simulink model "test"  (R2015a)
settings: Solver=ode1  StartTime=0.0  StopTime=10  FixedStep=0.001  RelTol=1e-3
PostLoadFcn:
  | , if any(exist('dsrtsu_mdlpostloadfcn', 'file') == [2, 3, 6]), try dsrtsu_mdlpostloadfcn('Execute', bdroot); catch fprintf('Error in PostLoadFcn (dsrtsu_mdlpostloadfcn) for model "%s":\n %s\n', bdroot, lasterr); end, end,
values from neighbouring files (symbols this model uses):
  c = rectangle('Parent',ax)    [DoublePendulum.m]    (also in init.m = 2.99880047981; interpolate.m = 2.99880047981; plot_17.m = 2.99880047981)
  g = 9.81    [init.m]    (also in interpolate.m; plot_17.m; plot_generic.m)
  T1 = 0.0395    [init.m]    (also in interpolate.m = 0.025; plot_17.m = 0.025; plot_generic.m)
settings Model: DSRTSU_INTERNAL_RTI_VER=360  DSRTSU_INTERNAL_RTI_TYPE=rti1104  CovSFcnEnable=off  Creator=labor  LastModifiedBy=Schuettler
settings DataIOCC: SignalLoggingSaveFormat=ModelDataLogs
settings OptimizationCC: BlockReduction=off  OptimizeBlockIOStorage=off  BufferReuse=off  GlobalBufferReuse=off  ExpressionFolding=off  ExpressionDepthLimit=2147483647  LocalBlockOutputs=off  InitFltsAndDblsToZero=on  OptimizeModelRefInitCode=on  LifeSpan=1
settings DebuggingCC: UnderspecifiedInitializationDetection=Classic  MergeDetectMultiDrivingBlocksExec=none  SolverPrmCheckMsg=warning  FcnCallInpInsideContextMsg=UseLocalSettings  StateNameClashWarn=warning
settings HardwareCC: ProdIntDivRoundTo=Zero  ProdEndianess=BigEndian  ProdHWDeviceType=Generic->Custom  TargetIntDivRoundTo=Zero  TargetEndianess=BigEndian  TargetHWDeviceType=Generic->Custom
settings RTWCC: SystemTargetFile=ert.tlc  TemplateMakefile=ert_default_tmf  Description=Embedded Coder
settings CodeAppCC: IgnoreCustomStorageClasses=off
settings ERTTargetCC: ParMdlRefBuildCompliant=on  CompOptLevelCompliant=on  ConcurrentExecutionCompliant=on  ERTFirstTimeCompliant=on  SupportContinuousTime=off  SupportVariableSizeSignals=off  ModelStepFunctionPrototypeControlCompliant=on  CPPClassGenCompliant=on  InlinedParameterPlacement=Hierarchical  ERTCustomFileTemplate=example_file_process.tlc

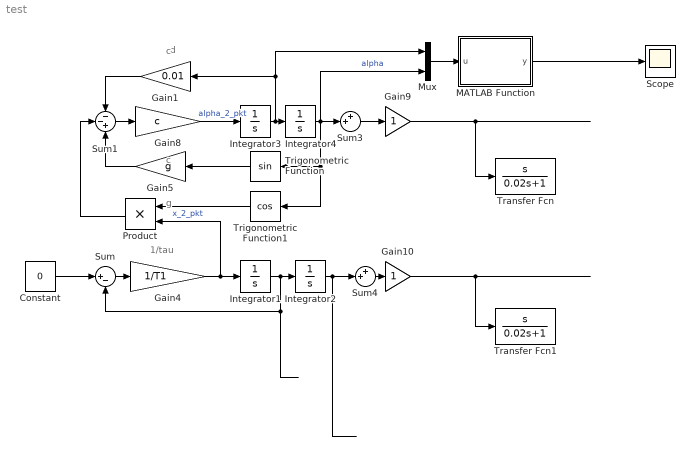
== system test ==
  note: d
  note: 1/tau
  note: g
  note: c
  note: c
  Constant : Constant  Value=0
  Gain1 : Gain  Gain=0.01
  Gain10 : Gain
  Gain4 : Gain  Gain=1/T1
  Gain5 : Gain  Gain=g
  Gain8 : Gain  Gain=c
  Gain9 : Gain
  Integrator1 : Integrator
  Integrator2 : Integrator
  Integrator3 : Integrator
  Integrator4 : Integrator  InitialCondition=2
  MATLAB Function : MATLAB Function  TreatAsAtomicUnit=on
  Mux : Mux  Inputs=2
  Product : Product  RndMeth=Zero
  Scope : Scope
      settings: SaveName=E
  Sum : Sum  Inputs=|+-
  Sum1 : Sum  Inputs=--+
  Sum3 : Sum  Inputs=++|
  Sum4 : Sum  Inputs=++|
  Transfer Fcn : TransferFcn  Numerator=[1 0]  Denominator=[0.02 1]
  Transfer Fcn1 : TransferFcn  Numerator=[1 0]  Denominator=[0.02 1]
  Trigonometric Function : Trigonometry
  Trigonometric Function1 : Trigonometry  Operator=cos
  wires:
  Sum3/1 -> Gain9/1
  Gain9/1 -> Transfer Fcn/1
  Gain10/1 -> Transfer Fcn1/1
  Sum4/1 -> Gain10/1
  Integrator1/1 -> Integrator2/1, Sum/2
  Integrator3/1 -> Gain1/1, Mux/1, Integrator4/1
  Gain4/1 -> Integrator1/1, Product/2  "x_2_pkt"
  Sum/1 -> Gain4/1
  Trigonometric Function1/1 -> Product/1
  Sum1/1 -> Gain8/1
  Gain8/1 -> Integrator3/1  "alpha_2_pkt"
  Integrator4/1 -> Mux/2, Sum3/2, Trigonometric Function/1, Trigonometric Function1/1  "alpha"
  Integrator2/1 -> Sum4/2
  Trigonometric Function/1 -> Gain5/1
  ? -> Sum3/1
  ? -> Sum4/1
  Gain5/1 -> Sum1/3
  Constant/1 -> Sum/1
  Product/1 -> Sum1/2
  Gain1/1 -> Sum1/1
  Mux/1 -> MATLAB Function/1(u)
  MATLAB Function/1(y) -> Scope/1

== matlab function test/MATLAB Function ==
  data: u input; y output
function y = fcn(u)

%g4 = 39.24;
g = 9.81;
l = 0.5;

%y = (u(1)^2*l + g4*(cos(u(2)) - 1))^2;
y = g*l/2*(cos(u(2))+1)+4*(l^2+0.002^2)/12*(u(1))^2/2;
